simulink model "model_1"  (R2021b)
settings: Solver=VariableStepAuto  StartTime=0.0  StopTime=5000  RelTol=1e-3
values from neighbouring files (symbols this model uses):
  A1 = [10, 7, 8; 2, 15, 10; 3, 11, 12]    [task_2.m]
  A2 = [0.5, 2, 0, 0; -2, 0.5, 0, 0; 0, 0, 0.3, 1; 0, 0, -1, 0.3]    [task_2.m]
  B1 = [1;2;3]    [task_2.m]
  B2 = zeros(3,4)    [task_2.m]
  C2 = [1, 1, 1]    [task_2.m]
  D2 = [1, -2, -1, -1]    [task_2.m]
  K1 = -Y1*inv(P1)    [task_2.m]
  K2 = Y2 - K1*P2    [task_2.m]
settings Model: Creator=vital  LastModifiedBy=vital

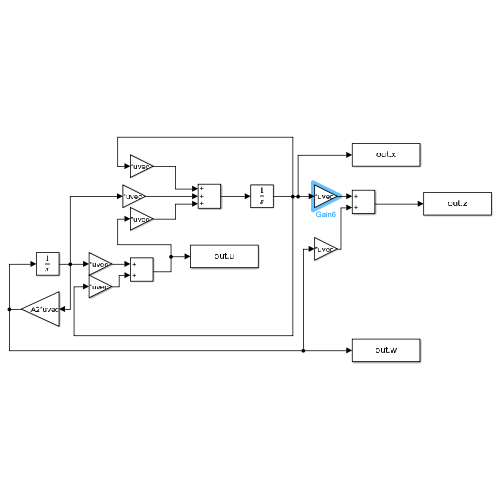
[thumbnail: Simulink's stored preview of the top-level diagram]
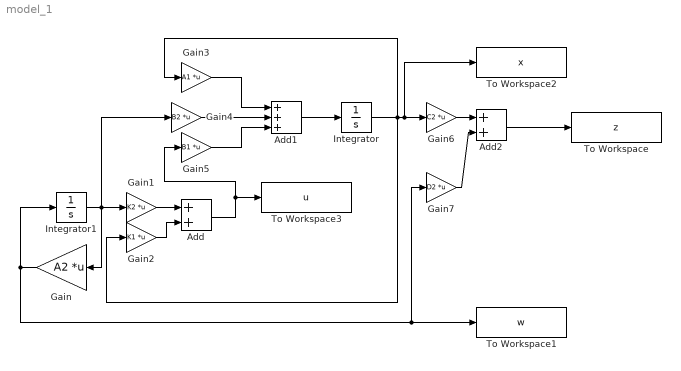
== system model_1 ==
  Add : Sum
  Add1 : Sum  Inputs=+++
  Add2 : Sum
  Gain : Gain  Gain=A2  Multiplication=Matrix(K*u) (u vector)
  Gain1 : Gain  Gain=K2  Multiplication=Matrix(K*u) (u vector)
  Gain2 : Gain  Gain=K1  Multiplication=Matrix(K*u) (u vector)
  Gain3 : Gain  Gain=A1  Multiplication=Matrix(K*u) (u vector)
  Gain4 : Gain  Gain=B2  Multiplication=Matrix(K*u) (u vector)
  Gain5 : Gain  Gain=B1  Multiplication=Matrix(K*u) (u vector)
  Gain6 : Gain  Gain=C2  Multiplication=Matrix(K*u) (u vector)
  Gain7 : Gain  Gain=D2  Multiplication=Matrix(K*u) (u vector)
  Integrator : Integrator
  Integrator1 : Integrator  InitialCondition=[1;1;1;1]
  To Workspace : ToWorkspace  VariableName=z  SaveFormat=Timeseries  SampleTime=-1
  To Workspace1 : ToWorkspace  VariableName=w  SaveFormat=Timeseries  SampleTime=-1
  To Workspace2 : ToWorkspace  VariableName=x  SaveFormat=Timeseries  SampleTime=-1
  To Workspace3 : ToWorkspace  VariableName=u  SaveFormat=Timeseries  SampleTime=-1
  wires:
  Integrator1/1 -> Gain4/1, Gain1/1, Gain/1
  Gain2/1 -> Add/2
  Gain1/1 -> Add/1
  Integrator/1 -> To Workspace2/1, Gain6/1, Gain3/1, Gain2/1
  Gain4/1 -> Add1/2
  Gain3/1 -> Add1/1
  Add/1 -> To Workspace3/1, Gain5/1
  Gain5/1 -> Add1/3
  Add1/1 -> Integrator/1
  Gain6/1 -> Add2/1
  Gain/1 -> Integrator1/1, To Workspace1/1, Gain7/1
  Gain7/1 -> Add2/2
  Add2/1 -> To Workspace/1
